simulink model "annotations"  (Simulink 6.3)
settings: Solver=ode45  StartTime=0.0  StopTime=50  RelTol=1e-3
settings Model: LastModifiedBy=deissenb

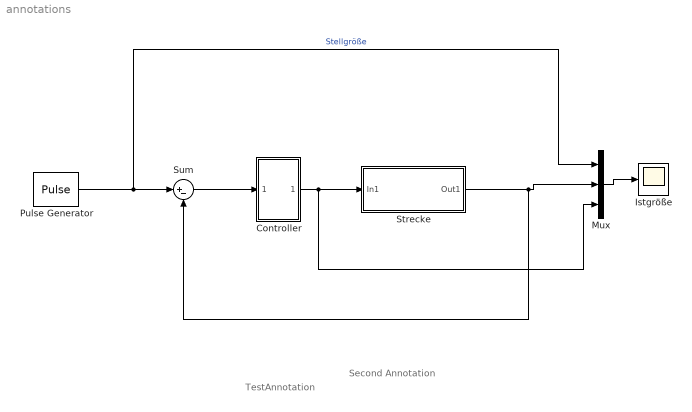
== system annotations ==
  note: TestAnnotation
  note: Second
      | Annotation
  Controller : Subsystem  TreatAsAtomicUnit=on  SystemSampleTime=[0.05,0]
  Istgröße : Scope
      settings: TimeRange=50  YMin=-2  YMax=2
  Mux : Mux  Inputs=3
  Pulse Generator : DiscretePulseGenerator  PulseType=Time based  PulseWidth=50
  Strecke : Subsystem
  Sum : Sum  Inputs=|+-
  wires:
  Pulse Generator/1 -> Sum/1, Mux/1  "Stellgröße"
  Strecke/1(Out1) -> Mux/2, Sum/2
  Mux/1 -> Istgröße/1
  Controller/1(Out1) -> Strecke/1(In1), Mux/3
  Sum/1 -> Controller/1(In1)

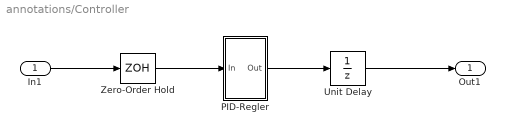
== system annotations/Controller ==
  In1 : Inport
  PID-Regler : Subsystem  TreatAsAtomicUnit=on
  Unit Delay : UnitDelay  SampleTime=-1
  Zero-Order Hold : ZeroOrderHold  SampleTime=-1
  Out1 : Outport
  wires:
  PID-Regler/1(Out) -> Unit Delay/1
  Zero-Order Hold/1 -> PID-Regler/1(In)
  In1/1 -> Zero-Order Hold/1
  Unit Delay/1 -> Out1/1

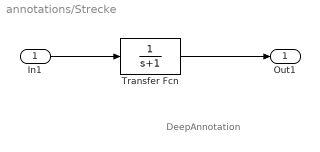
== system annotations/Strecke ==
  note: DeepAnnotation
  In1 : Inport
  Transfer Fcn : TransferFcn  Denominator=[1 1]
  Out1 : Outport
  wires:
  In1/1 -> Transfer Fcn/1
  Transfer Fcn/1 -> Out1/1

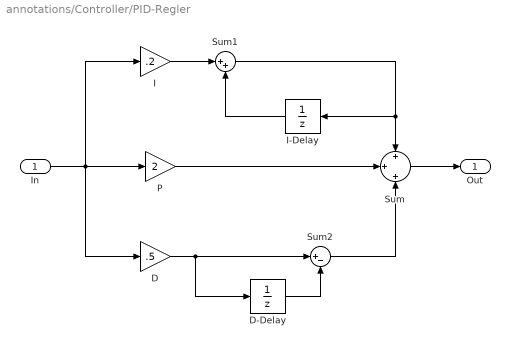
== system annotations/Controller/PID-Regler ==
  In : Inport
  D : Gain  Gain=.5
  D-Delay : UnitDelay  SampleTime=-1
  I : Gain  Gain=.2
  I-Delay : UnitDelay  Orientation=left  SampleTime=-1
  P : Gain  Gain=2
  Sum : Sum  Inputs=+|+|+
  Sum1 : Sum  Inputs=|++
  Sum2 : Sum  Inputs=|+-
  Out : Outport
  wires:
  P/1 -> Sum/2
  In/1 -> P/1, D/1, I/1
  Sum/1 -> Out/1
  I/1 -> Sum1/1
  Sum2/1 -> Sum/3
  Sum1/1 -> Sum/1, I-Delay/1
  D/1 -> Sum2/1, D-Delay/1
  D-Delay/1 -> Sum2/2
  I-Delay/1 -> Sum1/2
